simulink model "twoStoryBuildingDahldissertacaoJoao"  (R2017a)
settings: Solver=ode3  StartTime=0.0  StopTime=max(Time)  FixedStep=dt  RelTol=1e-3  EnableMultiTasking=on
values from neighbouring files (symbols this model uses):
  Kw = 57.42    [maincode.m]
  Kx = 0.7682    [maincode.m]
  rho = 27.45    [maincode.m]
undefined symbols (not defined in the file or in its folder): Ac, Bc, Cc, Dc, FlagSelect, x0
settings Model: Creator=Administrador  LastModifiedBy=vargas
settings DataIOCC: LimitDataPoints=on  SaveFormat=Array  SignalLoggingSaveFormat=ModelDataLogs
settings OptimizationCC: ExpressionDepthLimit=2147483647  LifeSpan=inf
settings DebuggingCC: UnderspecifiedInitializationDetection=Classic  MergeDetectMultiDrivingBlocksExec=none  SolverPrmCheckMsg=warning  FcnCallInpInsideContextMsg=warning  StateNameClashWarn=warning  SFUnexpectedBacktrackingDiag=warning  SFNoUnconditionalDefaultTransitionDiag=warning  SFExecutionAtInitializationDiag=none
settings HardwareCC: ProdBitPerPointer=32  ProdBitPerSizeT=32  ProdBitPerPtrDiffT=32  ProdLargestAtomicFloat=None  ProdIntDivRoundTo=Undefined  ProdEndianess=Unspecified  ProdWordSize=32  ProdHWDeviceType=32-bit Generic
settings ModelReferenceCC: PropagateSignalLabelsOutOfModel=off
settings GRTTargetCC: TargetLangStandard=C89/C90 (ANSI)  GeneratePreprocessorConditionals=Disable all  CombineOutputUpdateFcns=off  GRTInterface=on
settings ConfigComp: CovMetricSettings=dw  CovHtmlReporting=on  CovSaveCumulativeToWorkspaceVar=on  CovSaveSingleToWorkspaceVar=on  CovExternalEMLEnable=off

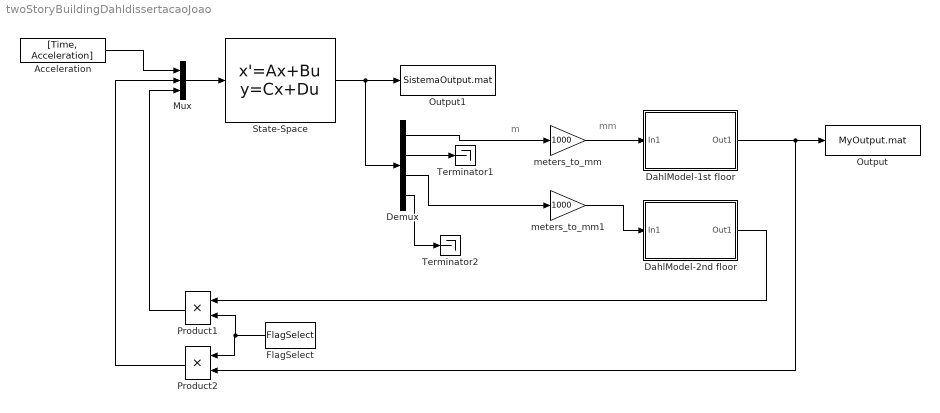
== system twoStoryBuildingDahldissertacaoJoao ==
  note: m
  note: mm
  Acceleration : FromWorkspace  VariableName=[Time, Acceleration]  SampleTime=0
  "DahlModel-1st floor " : Subsystem
  DahlModel-2nd floor : Subsystem
  Demux : Demux
  FlagSelect : Constant  Value=FlagSelect
  Mux : Mux  Inputs=3
  Output : ToFile  Filename=MyOutput.mat  MatrixName=MyOutput
  Output1 : ToFile  Filename=SistemaOutput.mat  MatrixName=SistemaOutput
  Product1 : Product  RndMeth=Zero
  Product2 : Product  RndMeth=Zero
  State-Space : StateSpace  A=Ac  B=Bc  C=Cc  D=Dc  X0=x0
  Terminator1 : Terminator
  Terminator2 : Terminator
  meters_to_mm : Gain  Gain=1000
  meters_to_mm1 : Gain  Gain=1000
  wires:
  Acceleration/1 -> Mux/1
  State-Space/1 -> Demux/1, Output1/1
  Mux/1 -> State-Space/1
  Demux/4 -> Terminator2/1
  "DahlModel-1st floor "/1(Out1) -> Product2/2, Output/1
  Demux/2 -> Terminator1/1
  FlagSelect/1 -> Product1/2, Product2/1
  Product2/1 -> Mux/2
  meters_to_mm/1 -> "DahlModel-1st floor "/1(In1)
  Demux/1 -> meters_to_mm/1
  Demux/3 -> meters_to_mm1/1
  meters_to_mm1/1 -> DahlModel-2nd floor/1(In1)
  DahlModel-2nd floor/1(Out1) -> Product1/1
  Product1/1 -> Mux/3

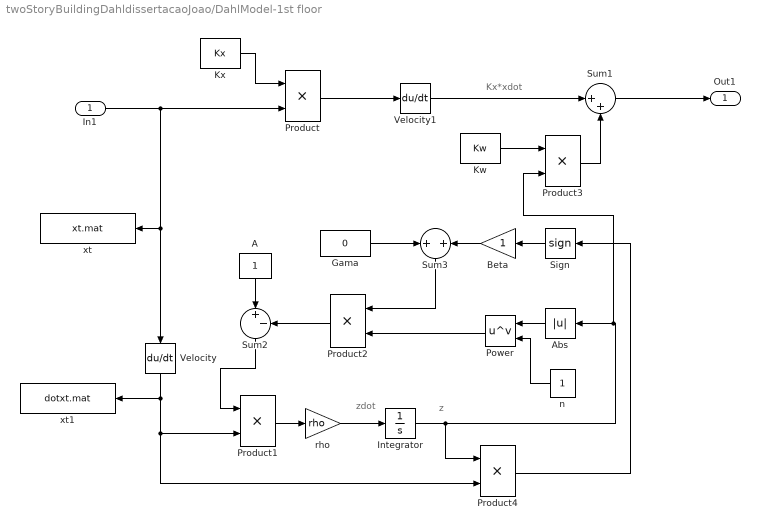
== system twoStoryBuildingDahldissertacaoJoao/DahlModel-1st floor  ==
  note: Kx*xdot
  note: zdot
  note: z
  In1 : Inport
  A : Constant
  Abs : Abs  SaturateOnIntegerOverflow=on
  Beta : Gain
  Gama : Constant  Value=0
  Integrator : Integrator
  Kw : Constant  Value=Kw
  Kx : Constant  Value=Kx
  Power : Math  Operator=pow  SaturateOnIntegerOverflow=on
  Product{,1..4} (5 alike) : Product  RndMeth=Zero
  Sign : Signum
  Sum1 : Sum  Inputs=|++
  Sum2 : Sum  Inputs=|+-
  Sum3 : Sum  Inputs=+|+
  Velocity : Derivative
  Velocity1 : Derivative
  n : Constant
  rho : Gain  Gain=rho
  xt : ToFile  Filename=xt.mat  MatrixName=xt
  xt1 : ToFile  Filename=dotxt.mat  MatrixName=dotxt
  Out1 : Outport
  wires:
  Power/1 -> Product2/2
  Product3/1 -> Sum1/2
  Sum1/1 -> Out1/1
  n/1 -> Power/2
  Abs/1 -> Power/1
  Kx/1 -> Product/1
  Velocity/1 -> Product4/2, Product1/2, xt1/1
  Sum2/1 -> Product1/1
  Product4/1 -> Sign/1
  Sign/1 -> Beta/1
  Beta/1 -> Sum3/2
  Gama/1 -> Sum3/1
  Sum3/1 -> Product2/1
  A/1 -> Sum2/1
  Product2/1 -> Sum2/2
  Product1/1 -> rho/1
  rho/1 -> Integrator/1
  Product/1 -> Velocity1/1
  Velocity1/1 -> Sum1/1
  Kw/1 -> Product3/1
  Integrator/1 -> Product4/1, Product3/2, Abs/1
  In1/1 -> xt/1, Velocity/1, Product/2

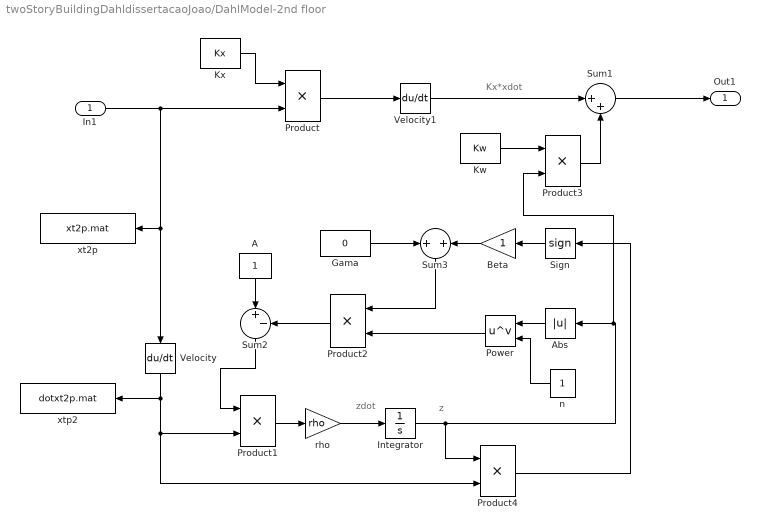
== system twoStoryBuildingDahldissertacaoJoao/DahlModel-2nd floor ==
  note: Kx*xdot
  note: zdot
  note: z
  In1 : Inport
  A : Constant
  Abs : Abs  SaturateOnIntegerOverflow=on
  Beta : Gain
  Gama : Constant  Value=0
  Integrator : Integrator
  Kw : Constant  Value=Kw
  Kx : Constant  Value=Kx
  Power : Math  Operator=pow  SaturateOnIntegerOverflow=on
  Product{,1..4} (5 alike) : Product  RndMeth=Zero
  Sign : Signum
  Sum1 : Sum  Inputs=|++
  Sum2 : Sum  Inputs=|+-
  Sum3 : Sum  Inputs=+|+
  Velocity : Derivative
  Velocity1 : Derivative
  n : Constant
  rho : Gain  Gain=rho
  xt2p : ToFile  Filename=xt2p.mat  MatrixName=xt2p
  xtp2 : ToFile  Filename=dotxt2p.mat  MatrixName=dotxt2p
  Out1 : Outport
  wires:
  Power/1 -> Product2/2
  Product3/1 -> Sum1/2
  Sum1/1 -> Out1/1
  n/1 -> Power/2
  Abs/1 -> Power/1
  Kx/1 -> Product/1
  Velocity/1 -> Product4/2, Product1/2, xtp2/1
  Sum2/1 -> Product1/1
  Product4/1 -> Sign/1
  Sign/1 -> Beta/1
  Beta/1 -> Sum3/2
  Gama/1 -> Sum3/1
  Sum3/1 -> Product2/1
  A/1 -> Sum2/1
  Product2/1 -> Sum2/2
  Product1/1 -> rho/1
  rho/1 -> Integrator/1
  Product/1 -> Velocity1/1
  Velocity1/1 -> Sum1/1
  Kw/1 -> Product3/1
  Integrator/1 -> Product4/1, Product3/2, Abs/1
  In1/1 -> xt2p/1, Velocity/1, Product/2
